simulink model "ex7l3"  (R2022b)
settings: Solver=VariableStepAuto  StartTime=0.0  StopTime=10.0  RelTol=1e-3
settings Model: Creator=gokuz  LastModifiedBy=gokuz

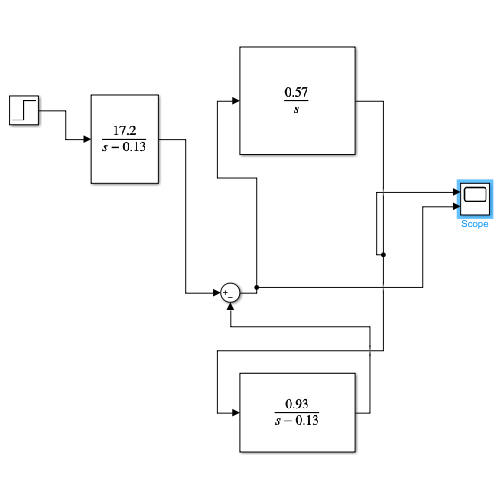
[thumbnail: Simulink's stored preview of the top-level diagram]
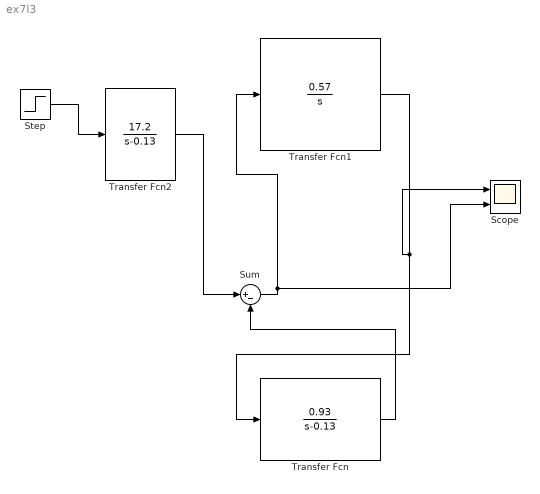
== system ex7l3 ==
  Scope : Scope  NumInputPorts=2
  Step : Step  SampleTime=0
  Sum : Sum  Inputs=|+-
  Transfer Fcn : TransferFcn  Numerator=[0 0.93]  Denominator=[1 -0.13]
  Transfer Fcn1 : TransferFcn  Numerator=[0 0.57]  Denominator=[1 0]
  Transfer Fcn2 : TransferFcn  Numerator=[0 17.2]  Denominator=[1 -0.13]
  wires:
  Step/1 -> Transfer Fcn2/1
  Transfer Fcn2/1 -> Sum/1
  Sum/1 -> Transfer Fcn1/1, Scope/2
  Transfer Fcn1/1 -> Transfer Fcn/1, Scope/1
  Transfer Fcn/1 -> Sum/2
